simulink model "psbmonophaseline"  (Simulink 6.0)
settings: Solver=ode23tb  SolverMode=SingleTasking  StartTime=0.0  StopTime=0.1  RelTol=1e-5  AbsTol=1e-5
libraries: powerlib2 x17
settings Model: Creator=patrice  LastModifiedBy=batserve  ExtModeTrigMode=oneshot  ExtModeArmWhenConnect=off  ExtModeAutoUpdateStatusClock=off
settings DataIOCC: LimitDataPoints=off  SaveOutput=off  SaveTime=off  SignalLoggingName=sigsOut
settings OptimizationCC: BlockReduction=off  BooleanDataType=off
settings DebuggingCC: CheckExecutionContextPreStartOutputMsg=on  CheckExecutionContextRuntimeOutputMsg=on  SolverPrmCheckMsg=none  IntegerOverflowMsg=none
settings HardwareCC: TargetUnknown=on
settings RTWCC: TemplateMakefile=grt_unix.tmf

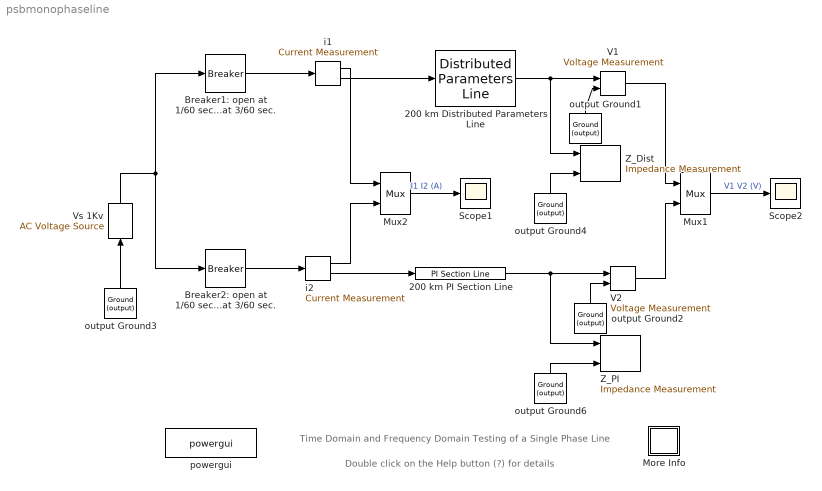
== system psbmonophaseline ==
  note: Time Domain and Frequency Domain Testing
      | of a Single Phase Line
  note: Double click on the Help button (?) for details
  200 km Distributed Parameters Line : powerlib2/Elements/Distributed Parameters Line  Tag=PoWeRsYsTeMbLoCk  n=1  f=60  r=0.0955  l=2.137e-3  c=12.37e-9  lgt=200  x1=[0 0 0 0; 0.0001244 0 0 0; 0.0002488 0 0 0; 0.0003733 0 0 0; 0.0004977 0 0 0; 0.0006221 0 0 0]  x2=[0 0 0 0; 0.0001244 0 0 0; 0.0002488 0 0 0; 0.0003733 0 0 0; 0.0004977 0 0 0; 0.0006221 0 0 0]  x3=[0 0 0 0; 0.0001244 0 0 0; 0.0002488 0 0 0; 0.0003733 0 0 0; 0.0004977 0 0 0; 0.0006221 0 0 0]  x4=[0 0 0 0; 0.0001244 0 0 0; 0.0002488 0 0 0; 0.0003733 0 0 0; 0.0004977 0 0 0; 0.0006221 0 0 0]  x5=0  mesure=None  PSBOutputType=111111111111111111111111111111
  200 km PI Section Line : powerlib2/Elements/PI Section Line  Tag=PoWeRsYsTeMbLoCk  f=60  a=0.0955  b=2.137e-03  c=12.37e-09  d=200  e=2  mesure=None  PSBOutputType=1
  Breaker1: open at 1/60 sec.  close at 3/60 sec. : powerlib2/Elements/Breaker  Tag=PoWeRsYsTeMbLoCk  a=0.1  c=1  rs=inf  cs=0  times="[ 1/60  3/60 ]"  Ts=0  comext=off  mesure=None  PSBOutputType=1
  Breaker2: open at 1/60 sec. close at 3/60 sec. : powerlib2/Elements/Breaker  Tag=PoWeRsYsTeMbLoCk  a=0.1  c=1  rs=inf  cs=0  times="[ 1/60  3/60 ]"  Ts=0  comext=off  mesure=None  PSBOutputType=1
  More Info : Subsystem
      mask Display: disp('?')
  Mux1 : Mux  Inputs=2
  Mux2 : Mux  Inputs=2
  Scope1 : Scope
      settings: TickLabels=on  TimeRange=0.1  YMin=-4  YMax=4  DataFormat=Array
  Scope2 : Scope
      settings: TickLabels=on  TimeRange=0.1  YMin=-2500  YMax=2500  DataFormat=Array
  V1 : powerlib2/Measurements/Voltage Measurement  Tag=PoWeRsYsTeMmEaSuReMeNt  PhasorSimulation=off  OutputType=Magnitude  PSBOutputType=0  PSBequivalent=0
  V2 : powerlib2/Measurements/Voltage Measurement  Tag=PoWeRsYsTeMmEaSuReMeNt  PhasorSimulation=off  OutputType=Magnitude  PSBOutputType=0  PSBequivalent=0
  Vs 1Kv : powerlib2/Electrical Sources/AC Voltage Source  Tag=PoWeRsYsTeMbLoCk  Orientation=up  A=1e3  P=0  F=60  stime=0  mesure=None  PSBOutputType=1
  Z_Dist : powerlib2/Measurements/Impedance Measurement  Tag=PoWeRsYsTeMbLoCk  kz=1
  Z_PI : powerlib2/Measurements/Impedance Measurement  Tag=PoWeRsYsTeMbLoCk  kz=1
  i1 : powerlib2/Measurements/Current Measurement  Tag=PoWeRsYsTeMmEaSuReMeNt  PhasorSimulation=off  OutputType=Magnitude  PSBOutputType=01  PSBequivalent=0
  i2 : powerlib2/Measurements/Current Measurement  Tag=PoWeRsYsTeMmEaSuReMeNt  PhasorSimulation=off  OutputType=Magnitude  PSBOutputType=01  PSBequivalent=0
  output Ground{1..4,6} (5 alike) : powerlib2/Connectors/Ground (output)  Tag=PoWeRsYsTeMbLoCk  Orientation=up  PSBOutputType=1
  powergui : powerlib2/powergui  Frange=0:2:2000  Ylog=on  Xlog=off  save=off  variable=ZData  ZoomFFT=on  StartTime=0.0  cycles=1  DisplayStyle=off  fundamental=60  FreqAxis=off  MaxFrequency=1000  frequencyindice=1  frequencyindicesteady=1  RmsSteady=1  display=on  Ts=0  methode=off  frequency=60  echomessages=off
  wires:
  Breaker1: open at 1/60 sec.  close at 3/60 sec./1 -> i1/1
  i1/2 -> 200 km Distributed Parameters Line/1
  output Ground1/1 -> V1/2
  i1/1 -> Mux2/1
  output Ground2/1 -> V2/2
  Breaker2: open at 1/60 sec. close at 3/60 sec./1 -> i2/1
  i2/2 -> 200 km PI Section Line/1
  i2/1 -> Mux2/2
  V1/1 -> Mux1/1
  V2/1 -> Mux1/2
  Mux1/1 -> Scope2/1  "V1 V2 (V)"
  output Ground3/1 -> Vs 1Kv/1
  Vs 1Kv/1 -> Breaker1: open at 1/60 sec.  close at 3/60 sec./1, Breaker2: open at 1/60 sec. close at 3/60 sec./1
  Mux2/1 -> Scope1/1  "I1 I2 (A)"
  200 km Distributed Parameters Line/1 -> V1/1, Z_Dist/1
  output Ground4/1 -> Z_Dist/2
  output Ground6/1 -> Z_PI/2
  200 km PI Section Line/1 -> V2/1, Z_PI/1

== system psbmonophaseline/More Info ==
  note: A  200 km line is connected on a 1 kV, 60 Hz  infinite source. The line is deenergized and then reenergized after 2 cycles.
      | The simulation is performed  simultaneously with two different line models:
      |
      | - Distributed parameter line
      | - PI  section line consisting of two 100 km sections.
      |
      | Currents at the sending end and voltages at the receiving end are compared for the two line models.
      | Impedance Measurement blocks are connected at the open end of both  lines in order  to compare their frequency responses.
  note: Open the two scopes and start the simulation.
      | Observe the difference in current and voltage waveforms at breaker opening and reclosing.
      | Note the sharp edges of the distributed parameter model (in yellow) .
      | These voltage and current steps which are due to travelling wave reflections at line ends are filtered by the PI model.
  note: Demonstration
  note: Circuit Description
  note: Open the Powergui block and select 'Steady-State Voltages and Currents' to display the voltage and current phasors.
      | Observe that the values obtained with the two models are the same.
  note: 2. Time domain comparison
  note: This demonstration compares time domain and frequencydomain performance
      | of distributed parameter line model and PI section line model
  note: 3. Frequency domain comparison
  note: Open  the Powergui block  and  select  'Impedance vs Frequency Measurement'.
      | A new window appears, listing the two Impedance Measurement blocks Z_Dist and Z_PI  connected to your circuit.
      | Note also that parameters are set to compute impedance in the 0:2000 Hz frequency range by steps of 2 Hz.
      | Using the 'CTRL' key, select both Z_Dist and Z_PI in the upper right window.
      | Then, click on the Display button.  The two impedances are computed and displayed on the same graph.
      |
      | Note that the distributed parameter line shows a succession of poles and zeros equally spaced, every 486 Hz.
      | The first pole occurs a 243 Hz , corresponding to frequency   f = 1 / (4*T)
      |
      | where :
      |
      |          T = travelling time = length*sqrt(L*C) = 200*sqrt(2.137e-3*12.37e-9) = 1.028 ms
      |
      | The PI section line only shows two poles because it consists of two PI sections.
      | Impedance comparison shows that a two-PI line gives a good approximation
      | of the distributed line for the 0-350 Hz frequency range.
  note: 1. Steady-state
  note: G. Sybille (Hydro-Quebec)
